simulink subsystem "MSD_DT_SS"  (R2022a)
settings: Solver=VariableStepAuto  StartTime=0.0  StopTime=10.0  RelTol=1e-3
values from neighbouring files (symbols this model uses):
  A_DT = SS_DT.A    [KalmanTesting_Mechanical.m]    (also in KalmanTesting_Mechanical_DataGeneration.m; KalmanTesting_Mechanical_InputQ_Sine.m; KalmanTesting_Mechanical_InputQ_Step.m; KalmanTesting_Mechanical_InputQ_Step_DataGen.m)
  B_DT = SS_DT.B    [KalmanTesting_Mechanical.m]    (also in KalmanTesting_Mechanical_DataGeneration.m; KalmanTesting_Mechanical_InputQ_Sine.m; KalmanTesting_Mechanical_InputQ_Step.m; KalmanTesting_Mechanical_InputQ_Step_DataGen.m)
  C = [1 1 1 1]    [KalmanTesting_Mechanical.m]    (also in KalmanTesting_Mechanical_DataGeneration.m = [0 0 0 1]; KalmanTesting_Mechanical_InputQ_Sine.m = [0 0 0 1]; KalmanTesting_Mechanical_InputQ_Step.m = [1 0 0 0]; KalmanTesting_Mechanical_InputQ_Step_DataGen.m = [0 0 0 1])
  Ts = 1    [KalmanTesting_Mechanical.m]    (also in KalmanTesting_Mechanical_DataGeneration.m = TT; KalmanTesting_Mechanical_InputQ_Sine.m = 1/SIM.fq/50; KalmanTesting_Mechanical_InputQ_Step.m = 0.1; KalmanTesting_Mechanical_InputQ_Step_DataGen.m = TT)
undefined symbols (not defined in the file or in its folder): x0
settings Model: Creator=tyevans  LastModifiedBy=tyevans

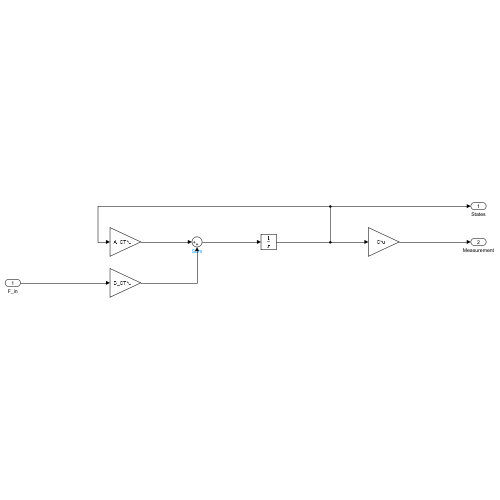
[thumbnail: Simulink's stored preview of the top-level diagram]
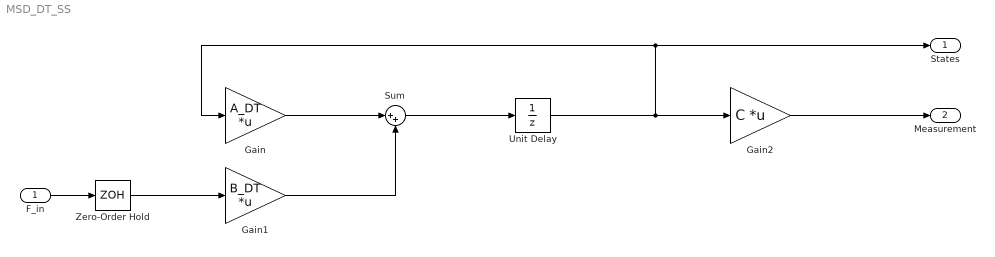
== system MSD_DT_SS ==
  F_in : Inport
  Gain : Gain  Gain=A_DT  Multiplication=Matrix(K*u)
  Gain1 : Gain  Gain=B_DT  Multiplication=Matrix(K*u)
  Gain2 : Gain  Gain=C  Multiplication=Matrix(K*u)
  Sum : Sum  Inputs=|++
  Unit Delay : UnitDelay  InitialCondition=x0  SampleTime=-1  HasFrameUpgradeWarning=on
  Zero-Order Hold : ZeroOrderHold  SampleTime=Ts
  States : Outport
  Measurement : Outport  Port=2
  wires:
  Unit Delay/1 -> Gain2/1, Gain/1, States/1
  Gain2/1 -> Measurement/1
  F_in/1 -> Zero-Order Hold/1
  Gain/1 -> Sum/1
  Sum/1 -> Unit Delay/1
  Gain1/1 -> Sum/2
  Zero-Order Hold/1 -> Gain1/1
